simulink model "Quaternions_Method_merge_main"  (R2021b)
settings: Solver=VariableStepAuto  StartTime=0.0  StopTime=Time  FixedStep=1e-1  RelTol=1e-13  AbsTol=1e-8
undefined symbols (not defined in the file or in its folder): a, A_BN_0, A_rw, A_rw_star, c, e, f_mag, H_0, i, magnitude, MB, mr, muP, omega_0, p_acc, RD, rho_d_MB, rho_s_MB, RS_MB, RS_SP, sig_b, sig_n, SP, T, t_sample, theta0, w_E
libraries: matrix_library x17, vrlib x8, simulink x2, simulink_extras x1
(part 4 of 6)

== system Quaternions_Method_merge_main/Sensors/Magnetometer1/Magnetometer /Error Matrices ==
  A_NonOrtho : Subsystem
  A_ScaleFactor : Subsystem
  A_eps : Subsystem
  A_no : Outport
  A_sf : Outport  Port=2
  A_noise : Outport  Port=3
  wires:
  A_NonOrtho/1(A_no) -> A_no/1
  A_ScaleFactor/1(A_sf) -> A_sf/1
  A_eps/1(A_eps) -> A_noise/1

== system Quaternions_Method_merge_main/Sensors/Magnetometer1/Magnetometer /RC Low Pass FIlter ==
  A* : Inport
  Add : Sum  Inputs=||+||-||
  Discrete Derivative : simulink/Discrete/Discrete Derivative  gainval=10  ICPrevScaledInput=0.0  OutMin=[]  OutMax=[]  OutDataType=fixdt(1, 16)  OutScaling=2^-10  DoSatur=off
  A*_filtered : Outport
  wires:
  A*/1 -> Add/1
  Add/1 -> Discrete Derivative/1, A*_filtered/1
  Discrete Derivative/1 -> Add/2

== system Quaternions_Method_merge_main/Sensors/Magnetometer1/Magnetometer /orthonormalization step 1 ==
  A*(t) : Inport
  Gain : Gain  Gain=3/2
  Gain1 : Gain  Gain=1/2
  Matrix Multiply : Product  Inputs=3  Multiplication=Matrix(*)
  Sum : Sum  Inputs=-+
  Transpose : Math  Operator=transpose  SaturateOnIntegerOverflow=on
  A_BN*_filtered : Outport
  wires:
  A*(t)/1 -> Transpose/1, Gain1/1, Matrix Multiply/1, Gain/1
  Sum/1 -> A_BN*_filtered/1
  Gain/1 -> Sum/2
  Transpose/1 -> Matrix Multiply/2
  Gain1/1 -> Matrix Multiply/3
  Matrix Multiply/1 -> Sum/1

== system Quaternions_Method_merge_main/Sensors/Magnetometer1/Magnetometer /orthonormalization step 2 ==
  A*(t) : Inport
  Gain : Gain  Gain=3/2
  Gain1 : Gain  Gain=1/2
  Matrix Multiply : Product  Inputs=3  Multiplication=Matrix(*)
  Sum : Sum  Inputs=-+
  Transpose : Math  Operator=transpose  SaturateOnIntegerOverflow=on
  A_BN*_filtered : Outport
  wires:
  Matrix Multiply/1 -> Sum/1
  Gain1/1 -> Matrix Multiply/3
  Transpose/1 -> Matrix Multiply/2
  Gain/1 -> Sum/2
  Sum/1 -> A_BN*_filtered/1
  A*(t)/1 -> Gain/1, Matrix Multiply/1, Gain1/1, Transpose/1

== system Quaternions_Method_merge_main/Sensors/Magnetometer1/Magnetometer /orthonormalization step 3 ==
  A*(t) : Inport
  Gain : Gain  Gain=3/2
  Gain1 : Gain  Gain=1/2
  Matrix Multiply : Product  Inputs=3  Multiplication=Matrix(*)
  Sum : Sum  Inputs=-+
  Transpose : Math  Operator=transpose  SaturateOnIntegerOverflow=on
  A_BN*_filtered : Outport
  wires:
  A*(t)/1 -> Transpose/1, Gain1/1, Matrix Multiply/1, Gain/1
  Sum/1 -> A_BN*_filtered/1
  Gain/1 -> Sum/2
  Transpose/1 -> Matrix Multiply/2
  Gain1/1 -> Matrix Multiply/3
  Matrix Multiply/1 -> Sum/1

== system Quaternions_Method_merge_main/Sensors/Magnetometer1/b_B computation/Saturation ==
  b_B : Inport
  Dot Product : DotProduct  InputSameDT=on  OutDataTypeStr=Inherit: Inherit via internal rule
  If : If  NumInputs=2  IfExpression=u1 < mr
  If Action Subsystem : Subsystem  TreatAsAtomicUnit=on
  If Action Subsystem1 : Subsystem  TreatAsAtomicUnit=on
  Merge : Merge
  Square Root : Sqrt  SaturateOnIntegerOverflow=on
  measurament range : Constant  Value=mr
  b_B saturated : Outport
  wires:
  b_B/1 -> If Action Subsystem1/2(b_B), Dot Product/2, If Action Subsystem/1(b_B), Dot Product/1
  Dot Product/1 -> Square Root/1
  If Action Subsystem/1(b_B*) -> Merge/1
  If/1 -> If Action Subsystem/Action
  If Action Subsystem1/1(b_B_sat) -> Merge/2
  If/2 -> If Action Subsystem1/Action
  Square Root/1 -> If/1
  measurament range/1 -> If Action Subsystem1/1(mr), If/2
  Merge/1 -> b_B saturated/1

== system Quaternions_Method_merge_main/Sun Pointing 1/Pointing error with quaternions/A_B_N from Euler to quaternion/Case 1 ==
  A11 : Inport
  A22 : Inport  Port=2
  A33 : Inport  Port=3
  Add : Sum  Inputs=++--
  Constant : Constant
  Gain : Gain  Gain=1/2
  Sqrt : Sqrt  SaturateOnIntegerOverflow=on
  q1 : Outport
  wires:
  A22/1 -> Add/3
  A11/1 -> Add/2
  A33/1 -> Add/4
  Constant/1 -> Add/1
  Add/1 -> Sqrt/1
  Sqrt/1 -> Gain/1
  Gain/1 -> q1/1

== system Quaternions_Method_merge_main/Sun Pointing 1/Pointing error with quaternions/A_B_N from Euler to quaternion/Case 2 ==
  A11 : Inport
  A22 : Inport  Port=2
  A33 : Inport  Port=3
  Add : Sum  Inputs=+-+-
  Constant : Constant
  Gain : Gain  Gain=1/2
  Sqrt : Sqrt  SaturateOnIntegerOverflow=on
  q2 : Outport
  wires:
  Gain/1 -> q2/1
  Sqrt/1 -> Gain/1
  Add/1 -> Sqrt/1
  Constant/1 -> Add/1
  A33/1 -> Add/4
  A11/1 -> Add/2
  A22/1 -> Add/3

== system Quaternions_Method_merge_main/Sun Pointing 1/Pointing error with quaternions/A_B_N from Euler to quaternion/Case 3 ==
  A11 : Inport
  A22 : Inport  Port=2
  A33 : Inport  Port=3
  Add : Sum  Inputs=+--+
  Constant : Constant
  Gain : Gain  Gain=1/2
  Sqrt : Sqrt  SaturateOnIntegerOverflow=on
  q3 : Outport
  wires:
  A22/1 -> Add/3
  A11/1 -> Add/2
  A33/1 -> Add/4
  Constant/1 -> Add/1
  Add/1 -> Sqrt/1
  Sqrt/1 -> Gain/1
  Gain/1 -> q3/1

== system Quaternions_Method_merge_main/Sun Pointing 1/Pointing error with quaternions/A_B_N from Euler to quaternion/Case 4 ==
  A11 : Inport
  A22 : Inport  Port=2
  A33 : Inport  Port=3
  Add : Sum  Inputs=++++
  Constant : Constant
  Gain : Gain  Gain=1/2
  Sqrt : Sqrt  SaturateOnIntegerOverflow=on
  q4 : Outport
  wires:
  Gain/1 -> q4/1
  Sqrt/1 -> Gain/1
  Add/1 -> Sqrt/1
  Constant/1 -> Add/1
  A33/1 -> Add/4
  A11/1 -> Add/2
  A22/1 -> Add/3

== system Quaternions_Method_merge_main/Sun Pointing 1/Pointing error with quaternions/A_B_N from Euler to quaternion/If Action Subsystem ==
  In2 : Inport
  In1 : Inport  Port=2
  Action Port : ActionPort  ActionPortLabel=if(u1 == u2)
  Add : Sum
  Add1 : Sum
  Add2 : Sum  Inputs=+-
  Demux : Demux  Outputs=6
  Gain : Gain  Gain=4
  Mux : Mux
  Product : Product
  Product1 : Product
  Product2 : Product
  Reciprocal : Product  Inputs=/
  Reshape : Reshape  OutputDimensionality=Column vector (2-D)
  q_vect1 : Outport
  wires:
  In1/1 -> Demux/1
  In2/1 -> [q1]
  Mux/1 -> Reshape/1
  Reshape/1 -> q_vect1/1
  [q1] -> Mux/1
  Demux/3 -> [A12]
  Demux/2 -> [A31]
  Demux/1 -> [A21]
  Demux/6 -> [A23]
  Demux/5 -> [A13]
  Demux/4 -> [A32]
  [q1] -> Gain/1
  Gain/1 -> Reciprocal/1
  Reciprocal/1 -> [q1_div]
  Add/1 -> Product/1
  [A21] -> Add/2
  [A12] -> Add/1
  [q1_div] -> Product/2
  Product/1 -> [q2]
  Product1/1 -> [q3]
  [q1_div] -> Product1/2
  [A13] -> Add1/1
  [A31] -> Add1/2
  Add1/1 -> Product1/1
  Add2/1 -> Product2/1
  [A32] -> Add2/2
  [A23] -> Add2/1
  [q1_div] -> Product2/2
  Product2/1 -> [q4]
  [q2] -> Mux/2
  [q3] -> Mux/3
  [q4] -> Mux/4

== system Quaternions_Method_merge_main/Sun Pointing 1/Pointing error with quaternions/A_B_N from Euler to quaternion/If Action Subsystem1 ==
  In2 : Inport
  In1 : Inport  Port=2
  Action Port : ActionPort  ActionPortLabel=elseif(u1 == u3)
  Add : Sum
  Add1 : Sum  Inputs=-+
  Add2 : Sum
  Demux : Demux  Outputs=6
  Gain : Gain  Gain=4
  Mux : Mux
  Product : Product
  Product1 : Product
  Product2 : Product
  Reciprocal : Product  Inputs=/
  Reshape : Reshape  OutputDimensionality=Column vector (2-D)
  q_vect2 : Outport
  wires:
  [q4] -> Mux/4
  [q3] -> Mux/3
  [q2] -> Mux/2
  Product2/1 -> [q3]
  [q2_div] -> Product2/2
  [A23] -> Add2/1
  [A32] -> Add2/2
  Add2/1 -> Product2/1
  Add1/1 -> Product1/1
  [A31] -> Add1/2
  [A13] -> Add1/1
  [q2_div] -> Product1/2
  Product1/1 -> [q4]
  Product/1 -> [q1]
  [q2_div] -> Product/2
  [A12] -> Add/1
  [A21] -> Add/2
  Add/1 -> Product/1
  Reciprocal/1 -> [q2_div]
  Gain/1 -> Reciprocal/1
  [q2] -> Gain/1
  Demux/4 -> [A32]
  Demux/5 -> [A13]
  Demux/6 -> [A23]
  Demux/1 -> [A21]
  Demux/2 -> [A31]
  Demux/3 -> [A12]
  [q1] -> Mux/1
  Reshape/1 -> q_vect2/1
  Mux/1 -> Reshape/1
  In2/1 -> [q2]
  In1/1 -> Demux/1

== system Quaternions_Method_merge_main/Sun Pointing 1/Pointing error with quaternions/A_B_N from Euler to quaternion/If Action Subsystem2 ==
  In2 : Inport
  In1 : Inport  Port=2
  Action Port : ActionPort  ActionPortLabel=elseif( u1 == u4)
  Add : Sum  Inputs=+-
  Add1 : Sum
  Add2 : Sum  Inputs=+-
  Demux : Demux  Outputs=6
  Gain : Gain  Gain=4
  Mux : Mux
  Product : Product
  Product1 : Product
  Product2 : Product
  Reciprocal : Product  Inputs=/
  Reshape : Reshape  OutputDimensionality=Column vector (2-D)
  q_vect3 : Outport
  wires:
  In1/1 -> Demux/1
  In2/1 -> [q3]
  Mux/1 -> Reshape/1
  Reshape/1 -> q_vect3/1
  [q1] -> Mux/1
  Demux/3 -> [A12]
  Demux/2 -> [A31]
  Demux/1 -> [A21]
  Demux/6 -> [A23]
  Demux/5 -> [A13]
  Demux/4 -> [A32]
  [q3] -> Gain/1
  Gain/1 -> Reciprocal/1
  Reciprocal/1 -> [q3_div]
  Add/1 -> Product/1
  [A21] -> Add/2
  [A12] -> Add/1
  [q3_div] -> Product/2
  Product/1 -> [q4]
  Product1/1 -> [q1]
  [q3_div] -> Product1/2
  [A13] -> Add1/1
  [A31] -> Add1/2
  Add1/1 -> Product1/1
  Add2/1 -> Product2/1
  [A32] -> Add2/2
  [A23] -> Add2/1
  [q3_div] -> Product2/2
  Product2/1 -> [q2]
  [q2] -> Mux/2
  [q3] -> Mux/3
  [q4] -> Mux/4

== system Quaternions_Method_merge_main/Sun Pointing 1/Pointing error with quaternions/A_B_N from Euler to quaternion/If Action Subsystem3 ==
  In2 : Inport
  In1 : Inport  Port=2
  Action Port : ActionPort  ActionPortLabel=elseif( u1 == u5)
  Add : Sum  Inputs=+-
  Add1 : Sum  Inputs=-+
  Add2 : Sum  Inputs=+-
  Demux : Demux  Outputs=6
  Gain : Gain  Gain=4
  Mux : Mux
  Product : Product
  Product1 : Product
  Product2 : Product
  Reciprocal : Product  Inputs=/
  Reshape : Reshape  OutputDimensionality=Column vector (2-D)
  q_vect4 : Outport
  wires:
  [q4] -> Mux/4
  [q3] -> Mux/3
  [q2] -> Mux/2
  Product2/1 -> [q1]
  [q4_div] -> Product2/2
  [A23] -> Add2/1
  [A32] -> Add2/2
  Add2/1 -> Product2/1
  Add1/1 -> Product1/1
  [A31] -> Add1/2
  [A13] -> Add1/1
  [q4_div] -> Product1/2
  Product1/1 -> [q2]
  Product/1 -> [q3]
  [q4_div] -> Product/2
  [A12] -> Add/1
  [A21] -> Add/2
  Add/1 -> Product/1
  Reciprocal/1 -> [q4_div]
  Gain/1 -> Reciprocal/1
  [q4] -> Gain/1
  Demux/4 -> [A32]
  Demux/5 -> [A13]
  Demux/6 -> [A23]
  Demux/1 -> [A21]
  Demux/2 -> [A31]
  Demux/3 -> [A12]
  [q1] -> Mux/1
  Reshape/1 -> q_vect4/1
  Mux/1 -> Reshape/1
  In2/1 -> [q4]
  In1/1 -> Demux/1

== system Quaternions_Method_merge_main/Sun Pointing 1/Pointing error with quaternions/A_B_N from attitude det to quaternion2/Case 1 ==
  A11 : Inport
  A22 : Inport  Port=2
  A33 : Inport  Port=3
  Add : Sum  Inputs=++--
  Constant : Constant
  Gain : Gain  Gain=1/2
  Sqrt : Sqrt  SaturateOnIntegerOverflow=on
  q1 : Outport
  wires:
  Gain/1 -> q1/1
  Sqrt/1 -> Gain/1
  Add/1 -> Sqrt/1
  Constant/1 -> Add/1
  A33/1 -> Add/4
  A11/1 -> Add/2
  A22/1 -> Add/3

== system Quaternions_Method_merge_main/Sun Pointing 1/Pointing error with quaternions/A_B_N from attitude det to quaternion2/Case 2 ==
  A11 : Inport
  A22 : Inport  Port=2
  A33 : Inport  Port=3
  Add : Sum  Inputs=+-+-
  Constant : Constant
  Gain : Gain  Gain=1/2
  Sqrt : Sqrt  SaturateOnIntegerOverflow=on
  q2 : Outport
  wires:
  A22/1 -> Add/3
  A11/1 -> Add/2
  A33/1 -> Add/4
  Constant/1 -> Add/1
  Add/1 -> Sqrt/1
  Sqrt/1 -> Gain/1
  Gain/1 -> q2/1

== system Quaternions_Method_merge_main/Sun Pointing 1/Pointing error with quaternions/A_B_N from attitude det to quaternion2/Case 3 ==
  A11 : Inport
  A22 : Inport  Port=2
  A33 : Inport  Port=3
  Add : Sum  Inputs=+--+
  Constant : Constant
  Gain : Gain  Gain=1/2
  Sqrt : Sqrt  SaturateOnIntegerOverflow=on
  q3 : Outport
  wires:
  Gain/1 -> q3/1
  Sqrt/1 -> Gain/1
  Add/1 -> Sqrt/1
  Constant/1 -> Add/1
  A33/1 -> Add/4
  A11/1 -> Add/2
  A22/1 -> Add/3

== system Quaternions_Method_merge_main/Sun Pointing 1/Pointing error with quaternions/A_B_N from attitude det to quaternion2/Case 4 ==
  A11 : Inport
  A22 : Inport  Port=2
  A33 : Inport  Port=3
  Add : Sum  Inputs=++++
  Constant : Constant
  Gain : Gain  Gain=1/2
  Sqrt : Sqrt  SaturateOnIntegerOverflow=on
  q4 : Outport
  wires:
  A22/1 -> Add/3
  A11/1 -> Add/2
  A33/1 -> Add/4
  Constant/1 -> Add/1
  Add/1 -> Sqrt/1
  Sqrt/1 -> Gain/1
  Gain/1 -> q4/1

== system Quaternions_Method_merge_main/Sun Pointing 1/Pointing error with quaternions/A_B_N from attitude det to quaternion2/If Action Subsystem ==
  In2 : Inport
  In1 : Inport  Port=2
  Action Port : ActionPort  ActionPortLabel=if(u1 == u2)
  Add : Sum
  Add1 : Sum
  Add2 : Sum  Inputs=+-
  Demux : Demux  Outputs=6
  Gain : Gain  Gain=4
  Mux : Mux
  Product : Product
  Product1 : Product
  Product2 : Product
  Reciprocal : Product  Inputs=/
  Reshape : Reshape  OutputDimensionality=Column vector (2-D)
  q_vect1 : Outport
  wires:
  [q4] -> Mux/4
  [q3] -> Mux/3
  [q2] -> Mux/2
  Product2/1 -> [q4]
  [q1_div] -> Product2/2
  [A23] -> Add2/1
  [A32] -> Add2/2
  Add2/1 -> Product2/1
  Add1/1 -> Product1/1
  [A31] -> Add1/2
  [A13] -> Add1/1
  [q1_div] -> Product1/2
  Product1/1 -> [q3]
  Product/1 -> [q2]
  [q1_div] -> Product/2
  [A12] -> Add/1
  [A21] -> Add/2
  Add/1 -> Product/1
  Reciprocal/1 -> [q1_div]
  Gain/1 -> Reciprocal/1
  [q1] -> Gain/1
  Demux/4 -> [A32]
  Demux/5 -> [A13]
  Demux/6 -> [A23]
  Demux/1 -> [A21]
  Demux/2 -> [A31]
  Demux/3 -> [A12]
  [q1] -> Mux/1
  Reshape/1 -> q_vect1/1
  Mux/1 -> Reshape/1
  In2/1 -> [q1]
  In1/1 -> Demux/1

== system Quaternions_Method_merge_main/Sun Pointing 1/Pointing error with quaternions/A_B_N from attitude det to quaternion2/If Action Subsystem1 ==
  In2 : Inport
  In1 : Inport  Port=2
  Action Port : ActionPort  ActionPortLabel=elseif(u1 == u3)
  Add : Sum
  Add1 : Sum  Inputs=-+
  Add2 : Sum
  Demux : Demux  Outputs=6
  Gain : Gain  Gain=4
  Mux : Mux
  Product : Product
  Product1 : Product
  Product2 : Product
  Reciprocal : Product  Inputs=/
  Reshape : Reshape  OutputDimensionality=Column vector (2-D)
  q_vect2 : Outport
  wires:
  In1/1 -> Demux/1
  In2/1 -> [q2]
  Mux/1 -> Reshape/1
  Reshape/1 -> q_vect2/1
  [q1] -> Mux/1
  Demux/3 -> [A12]
  Demux/2 -> [A31]
  Demux/1 -> [A21]
  Demux/6 -> [A23]
  Demux/5 -> [A13]
  Demux/4 -> [A32]
  [q2] -> Gain/1
  Gain/1 -> Reciprocal/1
  Reciprocal/1 -> [q2_div]
  Add/1 -> Product/1
  [A21] -> Add/2
  [A12] -> Add/1
  [q2_div] -> Product/2
  Product/1 -> [q1]
  Product1/1 -> [q4]
  [q2_div] -> Product1/2
  [A13] -> Add1/1
  [A31] -> Add1/2
  Add1/1 -> Product1/1
  Add2/1 -> Product2/1
  [A32] -> Add2/2
  [A23] -> Add2/1
  [q2_div] -> Product2/2
  Product2/1 -> [q3]
  [q2] -> Mux/2
  [q3] -> Mux/3
  [q4] -> Mux/4

== system Quaternions_Method_merge_main/Sun Pointing 1/Pointing error with quaternions/A_B_N from attitude det to quaternion2/If Action Subsystem2 ==
  In2 : Inport
  In1 : Inport  Port=2
  Action Port : ActionPort  ActionPortLabel=elseif( u1 == u4)
  Add : Sum  Inputs=+-
  Add1 : Sum
  Add2 : Sum  Inputs=+-
  Demux : Demux  Outputs=6
  Gain : Gain  Gain=4
  Mux : Mux
  Product : Product
  Product1 : Product
  Product2 : Product
  Reciprocal : Product  Inputs=/
  Reshape : Reshape  OutputDimensionality=Column vector (2-D)
  q_vect3 : Outport
  wires:
  [q4] -> Mux/4
  [q3] -> Mux/3
  [q2] -> Mux/2
  Product2/1 -> [q2]
  [q3_div] -> Product2/2
  [A23] -> Add2/1
  [A32] -> Add2/2
  Add2/1 -> Product2/1
  Add1/1 -> Product1/1
  [A31] -> Add1/2
  [A13] -> Add1/1
  [q3_div] -> Product1/2
  Product1/1 -> [q1]
  Product/1 -> [q4]
  [q3_div] -> Product/2
  [A12] -> Add/1
  [A21] -> Add/2
  Add/1 -> Product/1
  Reciprocal/1 -> [q3_div]
  Gain/1 -> Reciprocal/1
  [q3] -> Gain/1
  Demux/4 -> [A32]
  Demux/5 -> [A13]
  Demux/6 -> [A23]
  Demux/1 -> [A21]
  Demux/2 -> [A31]
  Demux/3 -> [A12]
  [q1] -> Mux/1
  Reshape/1 -> q_vect3/1
  Mux/1 -> Reshape/1
  In2/1 -> [q3]
  In1/1 -> Demux/1

== system Quaternions_Method_merge_main/Sun Pointing 1/Pointing error with quaternions/A_B_N from attitude det to quaternion2/If Action Subsystem3 ==
  In2 : Inport
  In1 : Inport  Port=2
  Action Port : ActionPort  ActionPortLabel=elseif( u1 == u5)
  Add : Sum  Inputs=+-
  Add1 : Sum  Inputs=-+
  Add2 : Sum  Inputs=+-
  Demux : Demux  Outputs=6
  Gain : Gain  Gain=4
  Mux : Mux
  Product : Product
  Product1 : Product
  Product2 : Product
  Reciprocal : Product  Inputs=/
  Reshape : Reshape  OutputDimensionality=Column vector (2-D)
  q_vect4 : Outport
  wires:
  In1/1 -> Demux/1
  In2/1 -> [q4]
  Mux/1 -> Reshape/1
  Reshape/1 -> q_vect4/1
  [q1] -> Mux/1
  Demux/3 -> [A12]
  Demux/2 -> [A31]
  Demux/1 -> [A21]
  Demux/6 -> [A23]
  Demux/5 -> [A13]
  Demux/4 -> [A32]
  [q4] -> Gain/1
  Gain/1 -> Reciprocal/1
  Reciprocal/1 -> [q4_div]
  Add/1 -> Product/1
  [A21] -> Add/2
  [A12] -> Add/1
  [q4_div] -> Product/2
  Product/1 -> [q3]
  Product1/1 -> [q2]
  [q4_div] -> Product1/2
  [A13] -> Add1/1
  [A31] -> Add1/2
  Add1/1 -> Product1/1
  Add2/1 -> Product2/1
  [A32] -> Add2/2
  [A23] -> Add2/1
  [q4_div] -> Product2/2
  Product2/1 -> [q1]
  [q2] -> Mux/2
  [q3] -> Mux/3
  [q4] -> Mux/4

== system Quaternions_Method_merge_main/Sun Pointing 1/Pointing error with quaternions/Desired attitude to quaternion1/Case 1 ==
  A11 : Inport
  A22 : Inport  Port=2
  A33 : Inport  Port=3
  Add : Sum  Inputs=++--
  Constant : Constant
  Gain : Gain  Gain=1/2
  Sqrt : Sqrt  SaturateOnIntegerOverflow=on
  q1 : Outport
  wires:
  A22/1 -> Add/3
  A11/1 -> Add/2
  A33/1 -> Add/4
  Constant/1 -> Add/1
  Add/1 -> Sqrt/1
  Sqrt/1 -> Gain/1
  Gain/1 -> q1/1

== system Quaternions_Method_merge_main/Sun Pointing 1/Pointing error with quaternions/Desired attitude to quaternion1/Case 2 ==
  A11 : Inport
  A22 : Inport  Port=2
  A33 : Inport  Port=3
  Add : Sum  Inputs=+-+-
  Constant : Constant
  Gain : Gain  Gain=1/2
  Sqrt : Sqrt  SaturateOnIntegerOverflow=on
  q2 : Outport
  wires:
  Gain/1 -> q2/1
  Sqrt/1 -> Gain/1
  Add/1 -> Sqrt/1
  Constant/1 -> Add/1
  A33/1 -> Add/4
  A11/1 -> Add/2
  A22/1 -> Add/3

== system Quaternions_Method_merge_main/Sun Pointing 1/Pointing error with quaternions/Desired attitude to quaternion1/Case 3 ==
  A11 : Inport
  A22 : Inport  Port=2
  A33 : Inport  Port=3
  Add : Sum  Inputs=+--+
  Constant : Constant
  Gain : Gain  Gain=1/2
  Sqrt : Sqrt  SaturateOnIntegerOverflow=on
  q3 : Outport
  wires:
  A22/1 -> Add/3
  A11/1 -> Add/2
  A33/1 -> Add/4
  Constant/1 -> Add/1
  Add/1 -> Sqrt/1
  Sqrt/1 -> Gain/1
  Gain/1 -> q3/1

== system Quaternions_Method_merge_main/Sun Pointing 1/Pointing error with quaternions/Desired attitude to quaternion1/Case 4 ==
  A11 : Inport
  A22 : Inport  Port=2
  A33 : Inport  Port=3
  Add : Sum  Inputs=++++
  Constant : Constant
  Gain : Gain  Gain=1/2
  Sqrt : Sqrt  SaturateOnIntegerOverflow=on
  q4 : Outport
  wires:
  Gain/1 -> q4/1
  Sqrt/1 -> Gain/1
  Add/1 -> Sqrt/1
  Constant/1 -> Add/1
  A33/1 -> Add/4
  A11/1 -> Add/2
  A22/1 -> Add/3

== system Quaternions_Method_merge_main/Sun Pointing 1/Pointing error with quaternions/Desired attitude to quaternion1/If Action Subsystem ==
  In2 : Inport
  In1 : Inport  Port=2
  Action Port : ActionPort  ActionPortLabel=if(u1 == u2)
  Add : Sum
  Add1 : Sum
  Add2 : Sum  Inputs=+-
  Demux : Demux  Outputs=6
  Gain : Gain  Gain=4
  Mux : Mux
  Product : Product
  Product1 : Product
  Product2 : Product
  Reciprocal : Product  Inputs=/
  Reshape : Reshape  OutputDimensionality=Column vector (2-D)
  q_vect1 : Outport
  wires:
  In1/1 -> Demux/1
  In2/1 -> [q1]
  Mux/1 -> Reshape/1
  Reshape/1 -> q_vect1/1
  [q1] -> Mux/1
  Demux/3 -> [A12]
  Demux/2 -> [A31]
  Demux/1 -> [A21]
  Demux/6 -> [A23]
  Demux/5 -> [A13]
  Demux/4 -> [A32]
  [q1] -> Gain/1
  Gain/1 -> Reciprocal/1
  Reciprocal/1 -> [q1_div]
  Add/1 -> Product/1
  [A21] -> Add/2
  [A12] -> Add/1
  [q1_div] -> Product/2
  Product/1 -> [q2]
  Product1/1 -> [q3]
  [q1_div] -> Product1/2
  [A13] -> Add1/1
  [A31] -> Add1/2
  Add1/1 -> Product1/1
  Add2/1 -> Product2/1
  [A32] -> Add2/2
  [A23] -> Add2/1
  [q1_div] -> Product2/2
  Product2/1 -> [q4]
  [q2] -> Mux/2
  [q3] -> Mux/3
  [q4] -> Mux/4

== system Quaternions_Method_merge_main/Sun Pointing 1/Pointing error with quaternions/Desired attitude to quaternion1/If Action Subsystem1 ==
  In2 : Inport
  In1 : Inport  Port=2
  Action Port : ActionPort  ActionPortLabel=elseif(u1 == u3)
  Add : Sum
  Add1 : Sum  Inputs=-+
  Add2 : Sum
  Demux : Demux  Outputs=6
  Gain : Gain  Gain=4
  Mux : Mux
  Product : Product
  Product1 : Product
  Product2 : Product
  Reciprocal : Product  Inputs=/
  Reshape : Reshape  OutputDimensionality=Column vector (2-D)
  q_vect2 : Outport
  wires:
  [q4] -> Mux/4
  [q3] -> Mux/3
  [q2] -> Mux/2
  Product2/1 -> [q3]
  [q2_div] -> Product2/2
  [A23] -> Add2/1
  [A32] -> Add2/2
  Add2/1 -> Product2/1
  Add1/1 -> Product1/1
  [A31] -> Add1/2
  [A13] -> Add1/1
  [q2_div] -> Product1/2
  Product1/1 -> [q4]
  Product/1 -> [q1]
  [q2_div] -> Product/2
  [A12] -> Add/1
  [A21] -> Add/2
  Add/1 -> Product/1
  Reciprocal/1 -> [q2_div]
  Gain/1 -> Reciprocal/1
  [q2] -> Gain/1
  Demux/4 -> [A32]
  Demux/5 -> [A13]
  Demux/6 -> [A23]
  Demux/1 -> [A21]
  Demux/2 -> [A31]
  Demux/3 -> [A12]
  [q1] -> Mux/1
  Reshape/1 -> q_vect2/1
  Mux/1 -> Reshape/1
  In2/1 -> [q2]
  In1/1 -> Demux/1

== system Quaternions_Method_merge_main/Sun Pointing 1/Pointing error with quaternions/Desired attitude to quaternion1/If Action Subsystem2 ==
  In2 : Inport
  In1 : Inport  Port=2
  Action Port : ActionPort  ActionPortLabel=elseif( u1 == u4)
  Add : Sum  Inputs=+-
  Add1 : Sum
  Add2 : Sum  Inputs=+-
  Demux : Demux  Outputs=6
  Gain : Gain  Gain=4
  Mux : Mux
  Product : Product
  Product1 : Product
  Product2 : Product
  Reciprocal : Product  Inputs=/
  Reshape : Reshape  OutputDimensionality=Column vector (2-D)
  q_vect3 : Outport
  wires:
  In1/1 -> Demux/1
  In2/1 -> [q3]
  Mux/1 -> Reshape/1
  Reshape/1 -> q_vect3/1
  [q1] -> Mux/1
  Demux/3 -> [A12]
  Demux/2 -> [A31]
  Demux/1 -> [A21]
  Demux/6 -> [A23]
  Demux/5 -> [A13]
  Demux/4 -> [A32]
  [q3] -> Gain/1
  Gain/1 -> Reciprocal/1
  Reciprocal/1 -> [q3_div]
  Add/1 -> Product/1
  [A21] -> Add/2
  [A12] -> Add/1
  [q3_div] -> Product/2
  Product/1 -> [q4]
  Product1/1 -> [q1]
  [q3_div] -> Product1/2
  [A13] -> Add1/1
  [A31] -> Add1/2
  Add1/1 -> Product1/1
  Add2/1 -> Product2/1
  [A32] -> Add2/2
  [A23] -> Add2/1
  [q3_div] -> Product2/2
  Product2/1 -> [q2]
  [q2] -> Mux/2
  [q3] -> Mux/3
  [q4] -> Mux/4

== system Quaternions_Method_merge_main/Sun Pointing 1/Pointing error with quaternions/Desired attitude to quaternion1/If Action Subsystem3 ==
  In2 : Inport
  In1 : Inport  Port=2
  Action Port : ActionPort  ActionPortLabel=elseif( u1 == u5)
  Add : Sum  Inputs=+-
  Add1 : Sum  Inputs=-+
  Add2 : Sum  Inputs=+-
  Demux : Demux  Outputs=6
  Gain : Gain  Gain=4
  Mux : Mux
  Product : Product
  Product1 : Product
  Product2 : Product
  Reciprocal : Product  Inputs=/
  Reshape : Reshape  OutputDimensionality=Column vector (2-D)
  q_vect4 : Outport
  wires:
  [q4] -> Mux/4
  [q3] -> Mux/3
  [q2] -> Mux/2
  Product2/1 -> [q1]
  [q4_div] -> Product2/2
  [A23] -> Add2/1
  [A32] -> Add2/2
  Add2/1 -> Product2/1
  Add1/1 -> Product1/1
  [A31] -> Add1/2
  [A13] -> Add1/1
  [q4_div] -> Product1/2
  Product1/1 -> [q2]
  Product/1 -> [q3]
  [q4_div] -> Product/2
  [A12] -> Add/1
  [A21] -> Add/2
  Add/1 -> Product/1
  Reciprocal/1 -> [q4_div]
  Gain/1 -> Reciprocal/1
  [q4] -> Gain/1
  Demux/4 -> [A32]
  Demux/5 -> [A13]
  Demux/6 -> [A23]
  Demux/1 -> [A21]
  Demux/2 -> [A31]
  Demux/3 -> [A12]
  [q1] -> Mux/1
  Reshape/1 -> q_vect4/1
  Mux/1 -> Reshape/1
  In2/1 -> [q4]
  In1/1 -> Demux/1

== system Quaternions_Method_merge_main/Enviroment/Solar Radiation Perturbation/Force/MB Forces/Dot Product N*MB ==
  S_B : Inport
  N_MB : Inport  Port=2
  Constant3 : Constant  Value=[1, 1, 1]
  Matrix Multiply5 : Product  Multiplication=Matrix(*)
  Product10 : Product
  Reshape11 : Reshape  OutputDimensionality=Row vector (2-D)
  Reshape12 : Reshape  OutputDimensionality=Column vector (2-D)
  Sum of Elements : Sum  Inputs=+  CollapseMode=Specified dimension  CollapseDim=2
  Out1 : Outport
  wires:
  N_MB/1 -> Product10/2
  Reshape11/1 -> Matrix Multiply5/1
  Constant3/1 -> Reshape11/1
  Matrix Multiply5/1 -> Product10/1
  Sum of Elements/1 -> Out1/1
  S_B/1 -> Reshape12/1
  Reshape12/1 -> Matrix Multiply5/2
  Product10/1 -> Sum of Elements/1

== system Quaternions_Method_merge_main/Enviroment/Solar Radiation Perturbation/Force/MB Forces/creation of the areas of the S//C ==
  note: creation of areas of MB:
      | a=lato corto su asse x del BF; b=lato lungo lungo asse y del BF; h = spessore lungo asse z del BF
  MB : Inport
  Demux : Demux
  Product1 : Product
  Product2 : Product
  Product4 : Product
  Terminator : Terminator
  a*b_1 : Outport
  a*b_2 : Outport  Port=2
  a*h_1 : Outport  Port=3
  a*h_2 : Outport  Port=4
  b*h_1 : Outport  Port=5
  b*h_2 : Outport  Port=6
  wires:
  Demux/4 -> Product4/1, Product2/2
  Demux/3 -> Product1/2, Product4/2
  Demux/2 -> Product1/1, Product2/1
  Product1/1 -> a*b_2/1, a*b_1/1  "a*b"
  Product2/1 -> a*h_1/1, a*h_2/1  "a*h"
  Product4/1 -> b*h_2/1, b*h_1/1  "b*h"
  MB/1 -> Demux/1
  Demux/1 -> Terminator/1

== system Quaternions_Method_merge_main/Enviroment/Solar Radiation Perturbation/Force/SP Forces/Dot Product N*SP ==
  S_B : Inport
  N_SP : Inport  Port=2
  Constant11 : Constant  Value=[1, 1, 1]
  Matrix Multiply7 : Product  Multiplication=Matrix(*)
  Product11 : Product
  Reshape13 : Reshape  OutputDimensionality=Column vector (2-D)
  Reshape8 : Reshape  OutputDimensionality=Row vector (2-D)
  Sum of Elements1 : Sum  Inputs=+  CollapseMode=Specified dimension  CollapseDim=2
  dot_N_SP_SB : Outport
  wires:
  Reshape13/1 -> Matrix Multiply7/2
  Matrix Multiply7/1 -> Product11/1
  N_SP/1 -> Product11/2
  Constant11/1 -> Reshape8/1
  Product11/1 -> Sum of Elements1/1
  Reshape8/1 -> Matrix Multiply7/1
  Sum of Elements1/1 -> dot_N_SP_SB/1
  S_B/1 -> Reshape13/1

== system Quaternions_Method_merge_main/Enviroment/Solar Radiation Perturbation/Force/SP Forces/creation of the areas of the S//C ==
  note: creation of areas of SP:
      | a=lato corto su asse x del BF; b=lato lungo lungo asse y del BF;
      | lato h è trascurabile
      | il procedimento è per 2 pannelli quindi in tutto ho 4 facce
  SP : Inport
  Demux1 : Demux
  Product1 : Product
  Terminator1 : Terminator
  Terminator3 : Terminator
  a*b_1 : Outport
  a*b_2 : Outport  Port=2
  a*b_3 : Outport  Port=3
  a*b_4 : Outport  Port=4
  wires:
  SP/1 -> Demux1/1
  Demux1/1 -> Terminator1/1
  Demux1/4 -> Terminator3/1
  Demux1/3 -> Product1/2
  Product1/1 -> a*b_3/1, a*b_1/1, a*b_4/1, a*b_2/1  "a*b"
  Demux1/2 -> Product1/1

== system Quaternions_Method_merge_main/Enviroment/Solar Radiation Perturbation/Sum forces/determine highlighted area/If Action Subsystem ==
  In1 : Inport
  Action Port : ActionPort  ActionPortLabel=if(u1>0 )
  Out1 : Outport
  wires:
  In1/1 -> Out1/1

== system Quaternions_Method_merge_main/Enviroment/Solar Radiation Perturbation/Sum forces/determine highlighted area/If Action Subsystem1 ==
  In1 : Inport
  Action Port : ActionPort  ActionPortLabel=elseif(u2>0)
  Out1 : Outport
  wires:
  In1/1 -> Out1/1

== system Quaternions_Method_merge_main/Enviroment/Solar Radiation Perturbation/Sum forces/determine highlighted area/If Action Subsystem2 ==
  Action Port : ActionPort  ActionPortLabel=else
  Constant : Constant  Value=0
  Out1 : Outport
  wires:
  Constant/1 -> Out1/1

== system Quaternions_Method_merge_main/Enviroment/Solar Radiation Perturbation/Sum forces/determine highlighted area/If Action Subsystem3 ==
  In1 : Inport
  Action Port : ActionPort  ActionPortLabel=if(u1>0 )
  Out1 : Outport
  wires:
  In1/1 -> Out1/1

== system Quaternions_Method_merge_main/Enviroment/Solar Radiation Perturbation/Sum forces/determine highlighted area/If Action Subsystem4 ==
  In1 : Inport
  Action Port : ActionPort  ActionPortLabel=elseif(u2>0)
  Out1 : Outport
  wires:
  In1/1 -> Out1/1

== system Quaternions_Method_merge_main/Enviroment/Solar Radiation Perturbation/Sum forces/determine highlighted area/If Action Subsystem5 ==
  Action Port : ActionPort  ActionPortLabel=else
  Constant : Constant  Value=0
  Out1 : Outport
  wires:
  Constant/1 -> Out1/1

== system Quaternions_Method_merge_main/Enviroment/Solar Radiation Perturbation/Sum forces/determine highlighted area/If Action Subsystem6 ==
  In1 : Inport
  Action Port : ActionPort  ActionPortLabel=if(u1>0 )
  Out1 : Outport
  wires:
  In1/1 -> Out1/1

== system Quaternions_Method_merge_main/Enviroment/Solar Radiation Perturbation/Sum forces/determine highlighted area/If Action Subsystem7 ==
  In1 : Inport
  Action Port : ActionPort  ActionPortLabel=elseif(u2>0)
  Out1 : Outport
  wires:
  In1/1 -> Out1/1

== system Quaternions_Method_merge_main/Enviroment/Solar Radiation Perturbation/Sum forces/determine highlighted area/If Action Subsystem8 ==
  Action Port : ActionPort  ActionPortLabel=else
  Constant : Constant  Value=0
  Out1 : Outport
  wires:
  Constant/1 -> Out1/1

== system Quaternions_Method_merge_main/Enviroment/Solar Radiation Perturbation/Sum forces/determine highlighted area/creazione della matrice che ha per colonne i vettori distanza tra il CM del MB e i centri geom delle aree illuminate dal sole  ==
  note: creo il vettore somma che ha per colonna i raggi vettori che collegano il CM del MB con i centri illuminati delle facce nel caso che il sole sia nelle 4 posizioni.
  MB : Inport
  A_vect : Inport  Port=2
  S_B : Inport  Port=3
  Gain : Gain  Gain=-1
  Gain1 : Gain  Gain=-1
  Gain2 : Gain  Gain=-1
  Reshape : Reshape  OutputDimensionality=Customize  OutputDimensions=[3,6]
  Transpose : Math  Operator=transpose  SaturateOnIntegerOverflow=on
  Vector Concatenate : Concatenate  NumInputs=6
  creazione raggi vettore tra CM MB e centro facce illuminate della faccia che ha come normale l'asse i : Subsystem
  creazione raggi vettore tra CM MB e centro facce illuminate della faccia che ha come normale l'asse j : Subsystem
  creazione raggi vettore tra CM MB e centro facce illuminate della faccia che ha come normale l'asse k : Subsystem
  distance matrix : Outport
  wires:
  creazione raggi vettore tra CM MB e centro facce illuminate della faccia che ha come normale l'asse k/1(Out1) -> Gain/1, Vector Concatenate/1
  Vector Concatenate/1 -> Reshape/1  "Areas k,-k,i,-i,j,-j"
  [S_B] -> creazione raggi vettore tra CM MB e centro facce illuminate della faccia che ha come normale l'asse k/1(S_B)
  [S_B] -> creazione raggi vettore tra CM MB e centro facce illuminate della faccia che ha come normale l'asse i/1(S_B)
  [S_B] -> creazione raggi vettore tra CM MB e centro facce illuminate della faccia che ha come normale l'asse j/1(S_B)
  A_vect/1 -> [A_vect]
  Gain/1 -> Vector Concatenate/2
  creazione raggi vettore tra CM MB e centro facce illuminate della faccia che ha come normale l'asse i/1(Out1) -> Gain1/1, Vector Concatenate/3
  Gain1/1 -> Vector Concatenate/4
  Gain2/1 -> Vector Concatenate/6
  creazione raggi vettore tra CM MB e centro facce illuminate della faccia che ha come normale l'asse j/1(Out1) -> Gain2/1, Vector Concatenate/5
  Reshape/1 -> Transpose/1
  Transpose/1 -> distance matrix/1
  MB/1 -> [MB]
  [MB] -> creazione raggi vettore tra CM MB e centro facce illuminate della faccia che ha come normale l'asse k/2(MB)
  [MB] -> creazione raggi vettore tra CM MB e centro facce illuminate della faccia che ha come normale l'asse i/2(MB)
  [MB] -> creazione raggi vettore tra CM MB e centro facce illuminate della faccia che ha come normale l'asse j/2(MB)
  [A_vect] -> creazione raggi vettore tra CM MB e centro facce illuminate della faccia che ha come normale l'asse k/3(A_vect)
  [A_vect] -> creazione raggi vettore tra CM MB e centro facce illuminate della faccia che ha come normale l'asse i/3(A_vect)
  [A_vect] -> creazione raggi vettore tra CM MB e centro facce illuminate della faccia che ha come normale l'asse j/3(A_vect)
  S_B/1 -> [S_B]

== system Quaternions_Method_merge_main/Enviroment/Solar Radiation Perturbation/Sum forces/determine highlighted area1/If Action Subsystem ==
  Action Port : ActionPort  ActionPortLabel=if(u1>0 )
  Constant : Constant  Value=[1;0]
  Out1 : Outport
  wires:
  Constant/1 -> Out1/1

== system Quaternions_Method_merge_main/Enviroment/Solar Radiation Perturbation/Sum forces/determine highlighted area1/If Action Subsystem1 ==
  Action Port : ActionPort  ActionPortLabel=elseif(u2>0)
  Constant : Constant  Value=[0;1]
  Out1 : Outport
  wires:
  Constant/1 -> Out1/1

== system Quaternions_Method_merge_main/Enviroment/Solar Radiation Perturbation/Sum forces/determine highlighted area1/If Action Subsystem2 ==
  Action Port : ActionPort  ActionPortLabel=else
  Constant : Constant  Value=[0;0]
  Out1 : Outport
  wires:
  Constant/1 -> Out1/1

== system Quaternions_Method_merge_main/Enviroment/Solar Radiation Perturbation/Sum forces/determine highlighted area1/If Action Subsystem3 ==
  Action Port : ActionPort  ActionPortLabel=if(u1>0 )
  Constant : Constant  Value=[1;0]
  Out1 : Outport
  wires:
  Constant/1 -> Out1/1

== system Quaternions_Method_merge_main/Enviroment/Solar Radiation Perturbation/Sum forces/determine highlighted area1/If Action Subsystem4 ==
  Action Port : ActionPort  ActionPortLabel=elseif(u2>0)
  Constant : Constant  Value=[0;1]
  Out1 : Outport
  wires:
  Constant/1 -> Out1/1

== system Quaternions_Method_merge_main/Enviroment/Solar Radiation Perturbation/Sum forces/determine highlighted area1/If Action Subsystem5 ==
  Action Port : ActionPort  ActionPortLabel=else
  Constant : Constant  Value=[0;0]
  Out1 : Outport
  wires:
  Constant/1 -> Out1/1

== system Quaternions_Method_merge_main/Enviroment/Solar Radiation Perturbation/Torque_arm/creazione raggi vettore tra CM MB e centro facce illuminate della faccia che ha come normale l'asse i/If Action Subsystem ==
  Areas_vect : Inport
  MB : Inport  Port=2
  Action Port : ActionPort  ActionPortLabel=if(u1>0 & u2>0)
  Add : Sum  Inputs=+|-
  Add1 : Sum  Inputs=+|-
  Add2 : Sum
  Demux : Demux  Outputs=3
  Demux2 : Demux
  Divide : Product  Inputs=*/
  Divide1 : Product  Inputs=*/
  Gain{,1..3} (4 alike) : Gain  Gain=1/2
  Ground : Ground
  Ground1 : Ground
  Mux : Mux  Inputs=3
  Mux1 : Mux  Inputs=3
  Reshape : Reshape  OutputDimensionality=Column vector (2-D)
  Reshape2 : Reshape  OutputDimensionality=Column vector (2-D)
  Reshape3 : Reshape  OutputDimensionality=Column vector (2-D)
  Terminator{1..2,8..9} (4 alike) : Terminator
  r_cface_cluce_yz_pos : Outport
  wires:
  Demux/2 -> Terminator8/1
  Demux/3 -> Terminator9/1
  Add2/1 -> r_cface_cluce_yz_pos/1
  Reshape3/1 -> Add2/2
  Reshape2/1 -> Add2/1
  [h_MB] -> Gain2/1
  Divide1/1 -> Gain3/1
  Gain2/1 -> Add1/1
  Gain3/1 -> Add1/2
  Ground/1 -> Mux1/2, Mux1/1
  Mux1/1 -> Reshape3/1  "raggio vettore che collega il centro geom della faccia con il centro geom della faccia illuminata dal sole lungo k"
  [b_MB] -> Divide1/2
  Reshape/1 -> Demux/1
  Ground1/1 -> Mux/3, Mux/1
  Areas_vect/1 -> Reshape/1
  [h_MB] -> Divide/2
  Gain/1 -> Add/1
  [b_MB] -> Gain/1
  Gain1/1 -> Add/2
  Mux/1 -> Reshape2/1  "raggio vettore che collega il centro geom della faccia con il centro geom della faccia illuminata dal sole lungo j"
  Divide/1 -> Gain1/1
  Demux/1 -> Divide1/1, Divide/1
  Add/1 -> Mux/2
  Add1/1 -> Mux1/3
  Demux2/1 -> Terminator2/1
  Demux2/2 -> Terminator1/1
  MB/1 -> Demux2/1
  Demux2/3 -> [b_MB]
  Demux2/4 -> [h_MB]

== system Quaternions_Method_merge_main/Enviroment/Solar Radiation Perturbation/Torque_arm/creazione raggi vettore tra CM MB e centro facce illuminate della faccia che ha come normale l'asse i/If Action Subsystem1 ==
  Areas_vect : Inport
  MB : Inport  Port=2
  Action Port : ActionPort  ActionPortLabel=if(u1>0 & u2<0)
  Add : Sum  Inputs=+|-
  Add1 : Sum  Inputs=+|-
  Add2 : Sum
  Demux : Demux  Outputs=3
  Demux2 : Demux
  Divide : Product  Inputs=*/
  Divide1 : Product  Inputs=*/
  Gain{,1..3} (4 alike) : Gain  Gain=1/2
  Gain4 : Gain  Gain=-1
  Ground : Ground
  Ground1 : Ground
  Mux : Mux  Inputs=3
  Mux1 : Mux  Inputs=3
  Reshape : Reshape  OutputDimensionality=Column vector (2-D)
  Reshape2 : Reshape  OutputDimensionality=Column vector (2-D)
  Reshape3 : Reshape  OutputDimensionality=Column vector (2-D)
  Terminator{1..2,8..9} (4 alike) : Terminator
  r_cface_cluce_yneg_z_pos : Outport
  wires:
  Add1/1 -> Mux1/3
  Demux/1 -> Divide/1, Divide1/1
  Divide/1 -> Gain1/1
  Mux/1 -> Reshape2/1  "raggio vettore che collega il centro geom della faccia con il centro geom della faccia illuminata dal sole lungo -j"
  Gain1/1 -> Add/2
  [b_MB] -> Gain/1
  Gain/1 -> Add/1
  [h_MB] -> Divide/2
  Areas_vect/1 -> Reshape/1
  Ground1/1 -> Mux/1, Mux/3
  Reshape/1 -> Demux/1
  [b_MB] -> Divide1/2
  Mux1/1 -> Reshape3/1  "raggio vettore che collega il centro geom della faccia con il centro geom della faccia illuminata dal sole lungo k"
  Ground/1 -> Mux1/1, Mux1/2
  Gain3/1 -> Add1/2
  Gain2/1 -> Add1/1
  Divide1/1 -> Gain3/1
  [h_MB] -> Gain2/1
  Reshape2/1 -> Add2/1
  Reshape3/1 -> Add2/2
  Add2/1 -> r_cface_cluce_yneg_z_pos/1
  Demux/3 -> Terminator9/1
  Demux/2 -> Terminator8/1
  Add/1 -> Gain4/1
  Gain4/1 -> Mux/2
  Demux2/1 -> Terminator2/1
  Demux2/2 -> Terminator1/1
  MB/1 -> Demux2/1
  Demux2/3 -> [b_MB]
  Demux2/4 -> [h_MB]

== system Quaternions_Method_merge_main/Enviroment/Solar Radiation Perturbation/Torque_arm/creazione raggi vettore tra CM MB e centro facce illuminate della faccia che ha come normale l'asse i/If Action Subsystem2 ==
  Areas_vect : Inport
  MB : Inport  Port=2
  Action Port : ActionPort  ActionPortLabel=if(u1<0 & u2<0)
  Add : Sum  Inputs=+|-
  Add1 : Sum  Inputs=+|-
  Add2 : Sum
  Demux : Demux  Outputs=3
  Demux2 : Demux
  Divide : Product  Inputs=*/
  Divide1 : Product  Inputs=*/
  Gain{,1..3} (4 alike) : Gain  Gain=1/2
  Gain4 : Gain  Gain=-1
  Gain5 : Gain  Gain=-1
  Ground : Ground
  Ground1 : Ground
  Mux : Mux  Inputs=3
  Mux1 : Mux  Inputs=3
  Reshape : Reshape  OutputDimensionality=Column vector (2-D)
  Reshape2 : Reshape  OutputDimensionality=Column vector (2-D)
  Reshape3 : Reshape  OutputDimensionality=Column vector (2-D)
  Terminator{1..2,8..9} (4 alike) : Terminator
  r_cface_cluce_yneg_z_neg : Outport
  wires:
  Gain4/1 -> Mux/2
  Add/1 -> Gain4/1
  Demux/2 -> Terminator8/1
  Demux/3 -> Terminator9/1
  Add2/1 -> r_cface_cluce_yneg_z_neg/1
  Reshape3/1 -> Add2/2
  Reshape2/1 -> Add2/1
  [h_MB] -> Gain2/1
  Divide1/1 -> Gain3/1
  Gain2/1 -> Add1/1
  Gain3/1 -> Add1/2
  Ground/1 -> Mux1/2, Mux1/1
  Mux1/1 -> Reshape3/1  "raggio vettore che collega il centro geom della faccia con il centro geom della faccia illuminata dal sole lungo -k"
  [b_MB] -> Divide1/2
  Reshape/1 -> Demux/1
  Ground1/1 -> Mux/3, Mux/1
  Areas_vect/1 -> Reshape/1
  [h_MB] -> Divide/2
  Gain/1 -> Add/1
  [b_MB] -> Gain/1
  Gain1/1 -> Add/2
  Mux/1 -> Reshape2/1  "raggio vettore che collega il centro geom della faccia con il centro geom della faccia illuminata dal sole lungo -j"
  Divide/1 -> Gain1/1
  Demux/1 -> Divide1/1, Divide/1
  Gain5/1 -> Mux1/3
  Add1/1 -> Gain5/1
  Demux2/1 -> Terminator2/1
  Demux2/2 -> Terminator1/1
  MB/1 -> Demux2/1
  Demux2/3 -> [b_MB]
  Demux2/4 -> [h_MB]

== system Quaternions_Method_merge_main/Enviroment/Solar Radiation Perturbation/Torque_arm/creazione raggi vettore tra CM MB e centro facce illuminate della faccia che ha come normale l'asse i/If Action Subsystem3 ==
  Action Port : ActionPort  ActionPortLabel=else
  Constant : Constant  Value=[0;0;0]
  Out1 : Outport
  wires:
  Constant/1 -> Out1/1

== system Quaternions_Method_merge_main/Enviroment/Solar Radiation Perturbation/Torque_arm/creazione raggi vettore tra CM MB e centro facce illuminate della faccia che ha come normale l'asse i/If Action Subsystem4 ==
  Areas_vect : Inport
  MB : Inport  Port=2
  Action Port : ActionPort  ActionPortLabel=if(u1<0 & u2>0)
  Add : Sum  Inputs=+|-
  Add1 : Sum  Inputs=+|-
  Add2 : Sum
  Demux : Demux  Outputs=3
  Demux2 : Demux
  Divide : Product  Inputs=*/
  Divide1 : Product  Inputs=*/
  Gain{,1..3} (4 alike) : Gain  Gain=1/2
  Gain4 : Gain  Gain=-1
  Ground : Ground
  Ground1 : Ground
  Mux : Mux  Inputs=3
  Mux1 : Mux  Inputs=3
  Reshape : Reshape  OutputDimensionality=Column vector (2-D)
  Reshape2 : Reshape  OutputDimensionality=Column vector (2-D)
  Reshape3 : Reshape  OutputDimensionality=Column vector (2-D)
  Terminator{1..2,8..9} (4 alike) : Terminator
  r_cface_cluce_zneg_y_pos : Outport
  wires:
  [h_MB] -> Divide1/2
  [b_MB] -> Gain2/1
  Add1/1 -> Mux1/2
  Gain4/1 -> Mux/3
  Add/1 -> Gain4/1
  [h_MB] -> Gain/1
  [b_MB] -> Divide/2
  Divide/1 -> Gain1/1
  Mux/1 -> Reshape2/1  "raggio vettore che collega il centro geom della faccia con il centro geom della faccia illuminata dal sole lungo -k"
  Gain1/1 -> Add/2
  Gain/1 -> Add/1
  Areas_vect/1 -> Reshape/1
  Ground1/1 -> Mux/1, Mux/2
  Reshape/1 -> Demux/1
  Mux1/1 -> Reshape3/1  "raggio vettore che collega il centro geom della faccia con il centro geom della faccia illuminata dal sole lungo j"
  Ground/1 -> Mux1/3, Mux1/1
  Gain3/1 -> Add1/2
  Gain2/1 -> Add1/1
  Divide1/1 -> Gain3/1
  Reshape2/1 -> Add2/1
  Reshape3/1 -> Add2/2
  Add2/1 -> r_cface_cluce_zneg_y_pos/1
  Demux/2 -> Terminator9/1
  Demux/3 -> Terminator8/1
  Demux/1 -> Divide1/1, Divide/1
  Demux2/1 -> Terminator2/1
  Demux2/2 -> Terminator1/1
  MB/1 -> Demux2/1
  Demux2/3 -> [b_MB]
  Demux2/4 -> [h_MB]

== system Quaternions_Method_merge_main/Enviroment/Solar Radiation Perturbation/Torque_arm/creazione raggi vettore tra CM MB e centro facce illuminate della faccia che ha come normale l'asse i/If Action Subsystem5 ==
  Action Port : ActionPort  ActionPortLabel=else
  Constant : Constant  Value=[0;0;0]
  Out1 : Outport
  wires:
  Constant/1 -> Out1/1

== system Quaternions_Method_merge_main/Enviroment/Solar Radiation Perturbation/Torque_arm/creazione raggi vettore tra CM MB e centro facce illuminate della faccia che ha come normale l'asse i/If Action Subsystem6 ==
  Action Port : ActionPort  ActionPortLabel=else
  Constant : Constant  Value=[0;0;0]
  Out1 : Outport
  wires:
  Constant/1 -> Out1/1

== system Quaternions_Method_merge_main/Enviroment/Solar Radiation Perturbation/Torque_arm/creazione raggi vettore tra CM MB e centro facce illuminate della faccia che ha come normale l'asse i/If Action Subsystem8 ==
  Action Port : ActionPort  ActionPortLabel=else
  Constant : Constant  Value=[0;0;0]
  Out1 : Outport
  wires:
  Constant/1 -> Out1/1

== system Quaternions_Method_merge_main/Enviroment/Solar Radiation Perturbation/Torque_arm/creazione raggi vettore tra CM MB e centro facce illuminate della faccia che ha come normale l'asse i/creating distance between cm MB and centro geom lato ==
  MB : Inport
  pointer : Inport  Port=2
  Demux : Demux
  Ground : Ground
  Mux : Mux  Inputs=3
  Product : Product
  Reshape : Reshape  OutputDimensionality=Column vector (2-D)
  Terminator : Terminator
  Terminator1 : Terminator
  Terminator3 : Terminator
  Out1 : Outport
  wires:
  Reshape/1 -> Out1/1
  Mux/1 -> Reshape/1
  MB/1 -> Demux/1
  Demux/1 -> Terminator/1
  Demux/2 -> Terminator1/1
  Ground/1 -> Mux/3, Mux/1
  Demux/4 -> Terminator3/1
  Demux/3 -> Product/1
  Product/1 -> Mux/2
  pointer/1 -> Product/2

== system Quaternions_Method_merge_main/Enviroment/Solar Radiation Perturbation/Torque_arm/creazione raggi vettore tra CM MB e centro facce illuminate della faccia che ha come normale l'asse j/If Action Subsystem ==
  Areas_vect : Inport
  MB : Inport  Port=2
  Action Port : ActionPort  ActionPortLabel=if(u1>0 & u2>0)
  Add : Sum  Inputs=+|-
  Add1 : Sum  Inputs=+|-
  Add2 : Sum
  Demux : Demux  Outputs=3
  Demux2 : Demux
  Divide : Product  Inputs=*/
  Divide1 : Product  Inputs=*/
  Gain{,1..3} (4 alike) : Gain  Gain=1/2
  Ground : Ground
  Ground1 : Ground
  Mux : Mux  Inputs=3
  Mux1 : Mux  Inputs=3
  Reshape : Reshape  OutputDimensionality=Column vector (2-D)
  Reshape2 : Reshape  OutputDimensionality=Column vector (2-D)
  Reshape3 : Reshape  OutputDimensionality=Column vector (2-D)
  Terminator{1..2,8..9} (4 alike) : Terminator
  r_cface_cluce_xz_pos : Outport
  wires:
  Add/1 -> Mux/3
  Divide/1 -> Gain1/1
  Mux/1 -> Reshape2/1  "raggio vettore che collega il centro geom della faccia con il centro geom della faccia illuminata dal sole lungo k"
  Gain1/1 -> Add/2
  Demux/2 -> Divide1/1, Divide/1
  [h_MB] -> Gain/1
  Gain/1 -> Add/1
  [a_MB] -> Divide/2
  Areas_vect/1 -> Reshape/1
  Ground1/1 -> Mux/2, Mux/1
  Reshape/1 -> Demux/1
  Add1/1 -> Mux1/1
  [h_MB] -> Divide1/2
  Mux1/1 -> Reshape3/1  "raggio vettore che collega il centro geom della faccia con il centro geom della faccia illuminata dal sole lungo i"
  Ground/1 -> Mux1/2, Mux1/3
  Gain3/1 -> Add1/2
  Gain2/1 -> Add1/1
  Divide1/1 -> Gain3/1
  [a_MB] -> Gain2/1
  Reshape2/1 -> Add2/1
  Reshape3/1 -> Add2/2
  Add2/1 -> r_cface_cluce_xz_pos/1
  Demux/1 -> Terminator9/1
  Demux/3 -> Terminator8/1
  Demux2/1 -> Terminator2/1
  Demux2/2 -> [a_MB]
  MB/1 -> Demux2/1
  Demux2/3 -> Terminator1/1
  Demux2/4 -> [h_MB]

== system Quaternions_Method_merge_main/Enviroment/Solar Radiation Perturbation/Torque_arm/creazione raggi vettore tra CM MB e centro facce illuminate della faccia che ha come normale l'asse j/If Action Subsystem1 ==
  Areas_vect : Inport
  MB : Inport  Port=2
  Action Port : ActionPort  ActionPortLabel=if(u1<0 & u2>0)
  Add : Sum  Inputs=+|-
  Add1 : Sum  Inputs=+|-
  Add2 : Sum
  Demux : Demux  Outputs=3
  Demux2 : Demux
  Divide : Product  Inputs=*/
  Divide1 : Product  Inputs=*/
  Gain{,1..3} (4 alike) : Gain  Gain=1/2
  Gain4 : Gain  Gain=-1
  Ground : Ground
  Ground1 : Ground
  Mux : Mux  Inputs=3
  Mux1 : Mux  Inputs=3
  Reshape : Reshape  OutputDimensionality=Column vector (2-D)
  Reshape2 : Reshape  OutputDimensionality=Column vector (2-D)
  Reshape3 : Reshape  OutputDimensionality=Column vector (2-D)
  Terminator{1..2,8..9} (4 alike) : Terminator
  r_cface_cluce_x_pos_z_neg : Outport
  wires:
  Demux/3 -> Terminator8/1
  Demux/1 -> Terminator9/1
  Add2/1 -> r_cface_cluce_x_pos_z_neg/1
  Reshape3/1 -> Add2/2
  Reshape2/1 -> Add2/1
  [a_MB] -> Gain2/1
  Divide1/1 -> Gain3/1
  Gain2/1 -> Add1/1
  Gain3/1 -> Add1/2
  Ground/1 -> Mux1/3, Mux1/2
  Mux1/1 -> Reshape3/1  "raggio vettore che collega il centro geom della faccia con il centro geom della faccia illuminata dal sole lungo i"
  [h_MB] -> Divide1/2
  Add1/1 -> Mux1/1
  Reshape/1 -> Demux/1
  Ground1/1 -> Mux/1, Mux/2
  Areas_vect/1 -> Reshape/1
  [a_MB] -> Divide/2
  Gain/1 -> Add/1
  [h_MB] -> Gain/1
  Demux/2 -> Divide/1, Divide1/1
  Gain1/1 -> Add/2
  Mux/1 -> Reshape2/1  "raggio vettore che collega il centro geom della faccia con il centro geom della faccia illuminata dal sole lungo -k"
  Divide/1 -> Gain1/1
  Add/1 -> Gain4/1
  Gain4/1 -> Mux/3
  Demux2/1 -> Terminator2/1
  Demux2/2 -> [a_MB]
  MB/1 -> Demux2/1
  Demux2/3 -> Terminator1/1
  Demux2/4 -> [h_MB]

== system Quaternions_Method_merge_main/Enviroment/Solar Radiation Perturbation/Torque_arm/creazione raggi vettore tra CM MB e centro facce illuminate della faccia che ha come normale l'asse j/If Action Subsystem2 ==
  Areas_vect : Inport
  MB : Inport  Port=2
  Action Port : ActionPort  ActionPortLabel=if(u1>0 & u2<0)
  Add : Sum  Inputs=+|-
  Add1 : Sum  Inputs=+|-
  Add2 : Sum
  Demux : Demux  Outputs=3
  Demux2 : Demux
  Divide : Product  Inputs=*/
  Divide1 : Product  Inputs=*/
  Gain{,1..3} (4 alike) : Gain  Gain=1/2
  Gain4 : Gain  Gain=-1
  Ground : Ground
  Ground1 : Ground
  Mux : Mux  Inputs=3
  Mux1 : Mux  Inputs=3
  Reshape : Reshape  OutputDimensionality=Column vector (2-D)
  Reshape2 : Reshape  OutputDimensionality=Column vector (2-D)
  Reshape3 : Reshape  OutputDimensionality=Column vector (2-D)
  Terminator{1..2,8..9} (4 alike) : Terminator
  r_cface_cluce_x_neg_z_pos : Outport
  wires:
  Add/1 -> Mux/3
  Divide/1 -> Gain1/1
  Mux/1 -> Reshape2/1  "raggio vettore che collega il centro geom della faccia con il centro geom della faccia illuminata dal sole lungo k"
  Gain1/1 -> Add/2
  Demux/2 -> Divide1/1, Divide/1
  [h_MB] -> Gain/1
  Gain/1 -> Add/1
  [a_MB] -> Divide/2
  Areas_vect/1 -> Reshape/1
  Ground1/1 -> Mux/2, Mux/1
  Reshape/1 -> Demux/1
  [h_MB] -> Divide1/2
  Mux1/1 -> Reshape3/1  "raggio vettore che collega il centro geom della faccia con il centro geom della faccia illuminata dal sole lungo -i"
  Ground/1 -> Mux1/2, Mux1/3
  Gain3/1 -> Add1/2
  Gain2/1 -> Add1/1
  Divide1/1 -> Gain3/1
  [a_MB] -> Gain2/1
  Reshape2/1 -> Add2/1
  Reshape3/1 -> Add2/2
  Add2/1 -> r_cface_cluce_x_neg_z_pos/1
  Demux/1 -> Terminator9/1
  Demux/3 -> Terminator8/1
  Gain4/1 -> Mux1/1
  Add1/1 -> Gain4/1
  Demux2/1 -> Terminator2/1
  Demux2/2 -> [a_MB]
  MB/1 -> Demux2/1
  Demux2/3 -> Terminator1/1
  Demux2/4 -> [h_MB]
